simulink model "FuelGaugingSystem"  (R2025a)
settings: Solver=ode23tb  StartTime=0.0  StopTime=1000  MaxStep=0.1  RelTol=1e-3
undefined symbols (not defined in the file): IN3_PER_GAL, KAPPA_NOMINAL
settings Model: DataDictionary=FuelGaugingData.sldd  Creator=mkelley  LastModifiedBy=mkelley

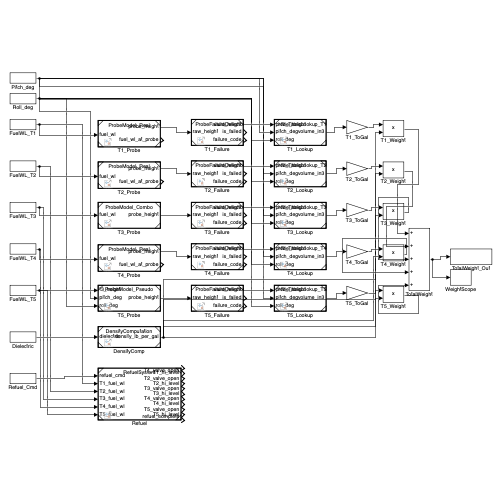
[thumbnail: Simulink's stored preview of the top-level diagram]
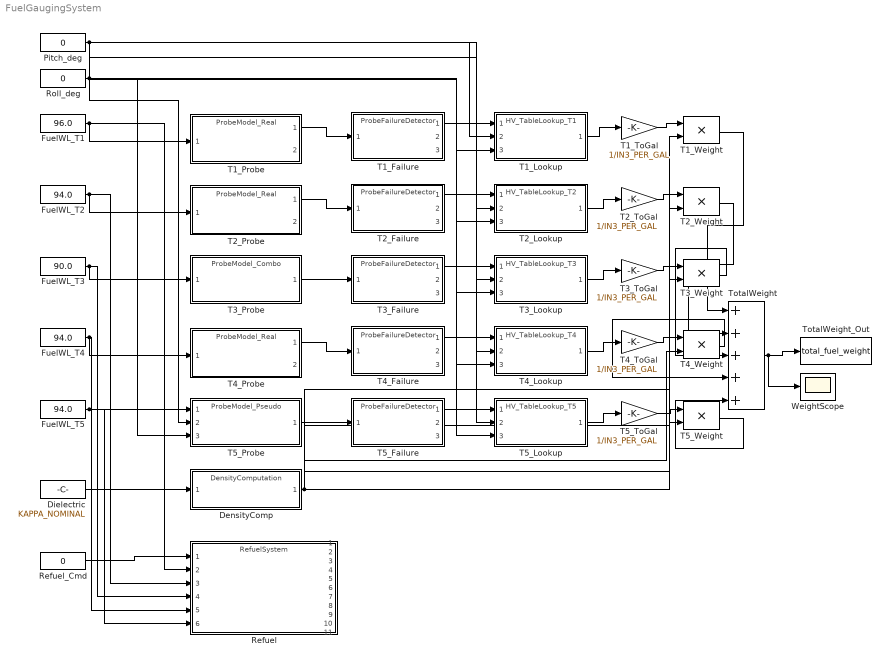
== system FuelGaugingSystem ==
  DensityComp : ModelReference  ModelNameDialog=DensityComputation  SimulationMode=Normal  ModelReferenceVersion=1.1
  Dielectric : Constant  Value=KAPPA_NOMINAL
  FuelWL_T1 : Constant  Value=96.0
  FuelWL_T2 : Constant  Value=94.0
  FuelWL_T3 : Constant  Value=90.0
  FuelWL_T4 : Constant  Value=94.0
  FuelWL_T5 : Constant  Value=94.0
  Pitch_deg : Constant  Value=0
  Refuel : ModelReference  ModelNameDialog=RefuelSystem  SimulationMode=Normal  ModelReferenceVersion=1.1
  Refuel_Cmd : Constant  Value=0
  Roll_deg : Constant  Value=0
  T1_Failure : ModelReference  ModelNameDialog=ProbeFailureDetector  SimulationMode=Normal  ModelReferenceVersion=1.1
  T1_Lookup : ModelReference  ModelNameDialog=HV_TableLookup_T1  SimulationMode=Normal  ModelReferenceVersion=1.1
  T1_Probe : ModelReference  ModelNameDialog=ProbeModel_Real  SimulationMode=Normal  ModelReferenceVersion=1.1
  T1_ToGal : Gain  Gain=1/IN3_PER_GAL
  T1_Weight : Product
  T2_Failure : ModelReference  ModelNameDialog=ProbeFailureDetector  SimulationMode=Normal  ModelReferenceVersion=1.1
  T2_Lookup : ModelReference  ModelNameDialog=HV_TableLookup_T2  SimulationMode=Normal  ModelReferenceVersion=1.1
  T2_Probe : ModelReference  ModelNameDialog=ProbeModel_Real  SimulationMode=Normal  ModelReferenceVersion=1.1
  T2_ToGal : Gain  Gain=1/IN3_PER_GAL
  T2_Weight : Product
  T3_Failure : ModelReference  ModelNameDialog=ProbeFailureDetector  SimulationMode=Normal  ModelReferenceVersion=1.1
  T3_Lookup : ModelReference  ModelNameDialog=HV_TableLookup_T3  SimulationMode=Normal  ModelReferenceVersion=1.1
  T3_Probe : ModelReference  ModelNameDialog=ProbeModel_Combo  SimulationMode=Normal  ModelReferenceVersion=1.1
  T3_ToGal : Gain  Gain=1/IN3_PER_GAL
  T3_Weight : Product
  T4_Failure : ModelReference  ModelNameDialog=ProbeFailureDetector  SimulationMode=Normal  ModelReferenceVersion=1.1
  T4_Lookup : ModelReference  ModelNameDialog=HV_TableLookup_T4  SimulationMode=Normal  ModelReferenceVersion=1.1
  T4_Probe : ModelReference  ModelNameDialog=ProbeModel_Real  SimulationMode=Normal  ModelReferenceVersion=1.1
  T4_ToGal : Gain  Gain=1/IN3_PER_GAL
  T4_Weight : Product
  T5_Failure : ModelReference  ModelNameDialog=ProbeFailureDetector  SimulationMode=Normal  ModelReferenceVersion=1.1
  T5_Lookup : ModelReference  ModelNameDialog=HV_TableLookup_T5  SimulationMode=Normal  ModelReferenceVersion=1.1
  T5_Probe : ModelReference  ModelNameDialog=ProbeModel_Pseudo  SimulationMode=Normal  ModelReferenceVersion=1.1
  T5_ToGal : Gain  Gain=1/IN3_PER_GAL
  T5_Weight : Product
  TotalWeight : Sum  Inputs=+++++
  TotalWeight_Out : ToWorkspace  VariableName=total_fuel_weight  SaveFormat=Timeseries  SampleTime=-1
  WeightScope : Scope
  wires:
  Dielectric/1 -> DensityComp/1
  Refuel_Cmd/1 -> Refuel/1
  FuelWL_T1/1 -> Refuel/2, T1_Probe/1
  FuelWL_T2/1 -> Refuel/3, T2_Probe/1
  FuelWL_T3/1 -> Refuel/4, T3_Probe/1
  FuelWL_T4/1 -> Refuel/5, T4_Probe/1
  FuelWL_T5/1 -> Refuel/6, T5_Probe/1
  T1_Probe/1 -> T1_Failure/1
  T1_Failure/1 -> T1_Lookup/1
  Pitch_deg/1 -> T1_Lookup/2, T2_Lookup/2, T3_Lookup/2, T4_Lookup/2, T5_Probe/2, T5_Lookup/2
  Roll_deg/1 -> T1_Lookup/3, T2_Lookup/3, T3_Lookup/3, T4_Lookup/3, T5_Probe/3, T5_Lookup/3
  T1_Lookup/1 -> T1_ToGal/1
  T1_ToGal/1 -> T1_Weight/1
  DensityComp/1 -> T1_Weight/2, T2_Weight/2, T3_Weight/2, T4_Weight/2, T5_Weight/2
  T1_Weight/1 -> TotalWeight/1
  T2_Probe/1 -> T2_Failure/1
  T2_Failure/1 -> T2_Lookup/1
  T2_Lookup/1 -> T2_ToGal/1
  T2_ToGal/1 -> T2_Weight/1
  T2_Weight/1 -> TotalWeight/2
  T3_Probe/1 -> T3_Failure/1
  T3_Failure/1 -> T3_Lookup/1
  T3_Lookup/1 -> T3_ToGal/1
  T3_ToGal/1 -> T3_Weight/1
  T3_Weight/1 -> TotalWeight/3
  T4_Probe/1 -> T4_Failure/1
  T4_Failure/1 -> T4_Lookup/1
  T4_Lookup/1 -> T4_ToGal/1
  T4_ToGal/1 -> T4_Weight/1
  T4_Weight/1 -> TotalWeight/4
  T5_Probe/1 -> T5_Failure/1
  T5_Failure/1 -> T5_Lookup/1
  T5_Lookup/1 -> T5_ToGal/1
  T5_ToGal/1 -> T5_Weight/1
  T5_Weight/1 -> TotalWeight/5
  TotalWeight/1 -> TotalWeight_Out/1, WeightScope/1
